simulink model "MesinAsinkronSatuFasa"  (R2017a)
settings: Solver=VariableStepAuto  StartTime=0.0  StopTime=10.0  RelTol=1e-3
libraries: powerlib x3
settings Model: Creator=Riza  LastModifiedBy=Riza

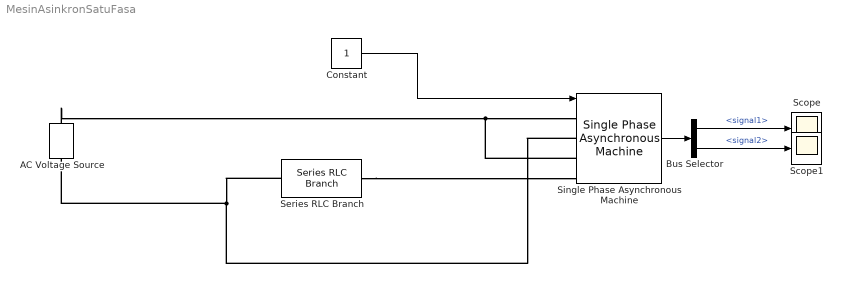
== system MesinAsinkronSatuFasa ==
  AC Voltage Source : powerlib/Electrical Sources/AC Voltage Source  Amplitude=100  Phase=0  Frequency=60  SampleTime=0  Measurements=None  BusType=swing  Pref=10e3  Qref=0  Qmin=-inf  Qmax=+inf
  Bus Selector : BusSelector  OutputSignals=signal1,signal2
  Constant : Constant
  Scope : Scope
  Scope1 : Scope
  Series RLC Branch : powerlib/Elements/Series RLC Branch  LConnTagsString=__new0  RConnTagsString=__new0  BranchType=RC  Resistance=1  Inductance=1e-3  SetiL0=off  InitialCurrent=0  Capacitance=1e-6  Setx0=off  InitialVoltage=0  Measurements=None
  Single Phase Asynchronous Machine : powerlib/Machines/Single Phase Asynchronous Machine  MechanicalLoad=Torque Tm  UNITS=SI  MachineType=Main & auxiliary windings  MeasurementBus=off  NominalParameters="[ .25*746  110  60]"  MainWindingStator="[2.02  7.4e-3]"  MainWindingRotor="[4.12  5.6e-3]"  MutualInductance=0.1772  AuxiliaryWinding="[7.14  8.5e-3]"  Mechanical="[0.0146  0  2 1.18]"  CapacitorStart="[2  254.7e-6]"  CapacitorRun="[18  21.1e-6]"  DisconnectionSpeed=75  InitialSpeed=0  DataType=SI  TsPowergui=0  TsBlock=-1
      settings: SourceProductName=Simscape Power Systems  SourceProductBaseCode=PS
  wires:
  Constant/1 -> Single Phase Asynchronous Machine/1
  Single Phase Asynchronous Machine/1 -> Bus Selector/1
  Bus Selector/1 -> Scope/1  "<signal1>"
  Bus Selector/2 -> Scope1/1  "<signal2>"
  connections:
  AC Voltage Source/RConn1 -- Single Phase Asynchronous Machine/LConn1 -- Single Phase Asynchronous Machine/LConn3
  Single Phase Asynchronous Machine/LConn2 -- Series RLC Branch/LConn1 -- AC Voltage Source/LConn1
  Series RLC Branch/RConn1 -- Single Phase Asynchronous Machine/LConn4
